simulink model "joystick"  (R2015a)
settings: Solver=ode45  StartTime=0.0  StopTime=inf  RelTol=1e-3
libraries: simulink x8, vrlib x1
settings Model: Creator=Trung Duc  LastModifiedBy=theth

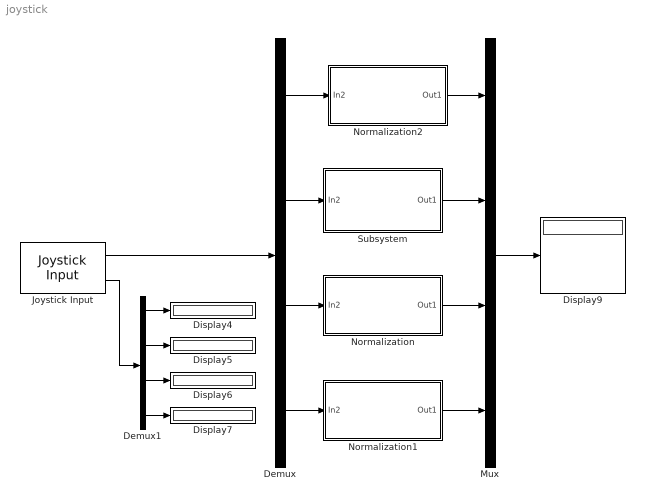
== system joystick ==
  Demux : Demux
  Demux1 : Demux
  Display{4..7,9} (5 alike) : Display
  Joystick Input : vrlib/Joystick Input  joyid=1  adjustports=on  forcefeed=off
  Mux : Mux
  Normalization : Subsystem
  Normalization1 : Subsystem
  Normalization2 : Subsystem
  Subsystem : Subsystem
  wires:
  Joystick Input/1 -> Demux/1
  Demux/1 -> Normalization2/1(In2)
  Demux1/1 -> Display4/1
  Demux1/2 -> Display5/1
  Demux1/3 -> Display6/1
  Demux1/4 -> Display7/1
  Joystick Input/2 -> Demux1/1
  Normalization2/1(Out1) -> Mux/1
  Normalization1/1(Out1) -> Mux/4
  Mux/1 -> Display9/1
  Demux/3 -> Normalization/1(In2)
  Normalization/1(Out1) -> Mux/3
  Demux/4 -> Normalization1/1(In2)
  Demux/2 -> Subsystem/1(In2)
  Subsystem/1(Out1) -> Mux/2

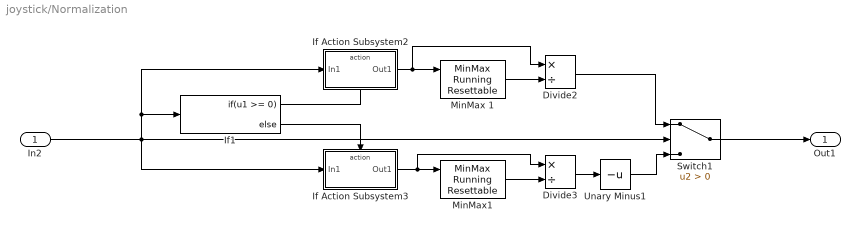
== system joystick/Normalization ==
  In2 : Inport
  Divide2 : Product  Inputs=*/
  Divide3 : Product  Inputs=*/
  If Action Subsystem2 : Subsystem  TreatAsAtomicUnit=on
  If Action Subsystem3 : Subsystem  TreatAsAtomicUnit=on
  If1 : If  IfExpression=u1 >= 0
  MinMax 1 : simulink/Math Operations/MinMax Running Resettable  Function=max  vinit=0.0
  MinMax1 : simulink/Math Operations/MinMax Running Resettable  Function=min  vinit=0.0
  Switch1 : Switch  Criteria=u2 > Threshold
  Unary Minus1 : UnaryMinus
  Out1 : Outport
  wires:
  Divide2/1 -> Switch1/1
  MinMax 1/1 -> Divide2/2
  If Action Subsystem2/1(Out1) -> Divide2/1, MinMax 1/1
  If1/1 -> If Action Subsystem2/Action
  Switch1/1 -> Out1/1
  If Action Subsystem3/1(Out1) -> MinMax1/1, Divide3/1
  MinMax1/1 -> Divide3/2
  In2/1 -> If Action Subsystem3/1(In1), Switch1/2, If Action Subsystem2/1(In1), If1/1
  Unary Minus1/1 -> Switch1/3
  Divide3/1 -> Unary Minus1/1
  If1/2 -> If Action Subsystem3/Action

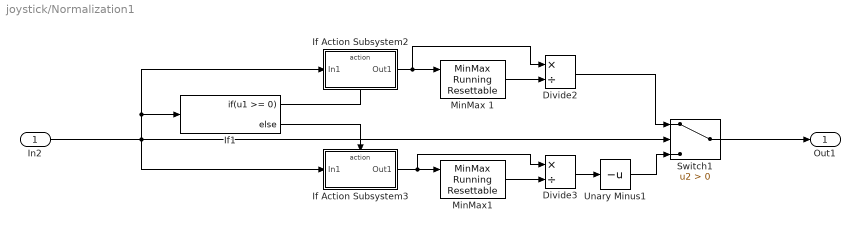
== system joystick/Normalization1 ==
  In2 : Inport
  Divide2 : Product  Inputs=*/
  Divide3 : Product  Inputs=*/
  If Action Subsystem2 : Subsystem  TreatAsAtomicUnit=on
  If Action Subsystem3 : Subsystem  TreatAsAtomicUnit=on
  If1 : If  IfExpression=u1 >= 0
  MinMax 1 : simulink/Math Operations/MinMax Running Resettable  Function=max  vinit=0.0
  MinMax1 : simulink/Math Operations/MinMax Running Resettable  Function=min  vinit=0.0
  Switch1 : Switch  Criteria=u2 > Threshold
  Unary Minus1 : UnaryMinus
  Out1 : Outport
  wires:
  Divide2/1 -> Switch1/1
  MinMax 1/1 -> Divide2/2
  If Action Subsystem2/1(Out1) -> Divide2/1, MinMax 1/1
  If1/1 -> If Action Subsystem2/Action
  Switch1/1 -> Out1/1
  If Action Subsystem3/1(Out1) -> MinMax1/1, Divide3/1
  MinMax1/1 -> Divide3/2
  In2/1 -> If Action Subsystem3/1(In1), Switch1/2, If Action Subsystem2/1(In1), If1/1
  Unary Minus1/1 -> Switch1/3
  Divide3/1 -> Unary Minus1/1
  If1/2 -> If Action Subsystem3/Action

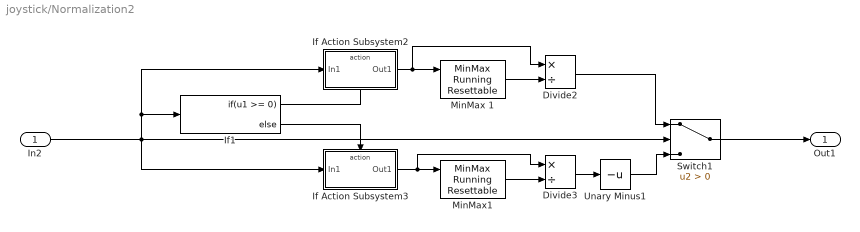
== system joystick/Normalization2 ==
  In2 : Inport
  Divide2 : Product  Inputs=*/
  Divide3 : Product  Inputs=*/
  If Action Subsystem2 : Subsystem  TreatAsAtomicUnit=on
  If Action Subsystem3 : Subsystem  TreatAsAtomicUnit=on
  If1 : If  IfExpression=u1 >= 0
  MinMax 1 : simulink/Math Operations/MinMax Running Resettable  Function=max  vinit=0.0
  MinMax1 : simulink/Math Operations/MinMax Running Resettable  Function=min  vinit=0.0
  Switch1 : Switch  Criteria=u2 > Threshold
  Unary Minus1 : UnaryMinus
  Out1 : Outport
  wires:
  Divide2/1 -> Switch1/1
  MinMax 1/1 -> Divide2/2
  If Action Subsystem2/1(Out1) -> Divide2/1, MinMax 1/1
  If1/1 -> If Action Subsystem2/Action
  Switch1/1 -> Out1/1
  If Action Subsystem3/1(Out1) -> MinMax1/1, Divide3/1
  MinMax1/1 -> Divide3/2
  In2/1 -> If Action Subsystem3/1(In1), Switch1/2, If Action Subsystem2/1(In1), If1/1
  Unary Minus1/1 -> Switch1/3
  Divide3/1 -> Unary Minus1/1
  If1/2 -> If Action Subsystem3/Action

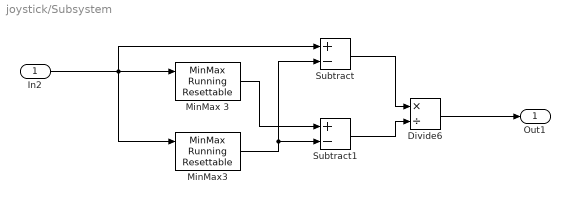
== system joystick/Subsystem ==
  In2 : Inport
  Divide6 : Product  Inputs=*/
  MinMax 3 : simulink/Math Operations/MinMax Running Resettable  Function=max  vinit=0.0
  MinMax3 : simulink/Math Operations/MinMax Running Resettable  Function=min  vinit=0.0
  Subtract : Sum  Inputs=+-
  Subtract1 : Sum  Inputs=+-
  Out1 : Outport
  wires:
  MinMax 3/1 -> Subtract1/1
  Subtract1/1 -> Divide6/2
  Divide6/1 -> Out1/1
  MinMax3/1 -> Subtract/2, Subtract1/2
  Subtract/1 -> Divide6/1
  In2/1 -> MinMax 3/1, MinMax3/1, Subtract/1

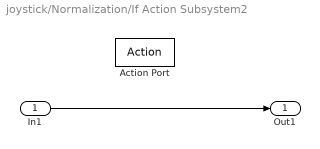
== system joystick/Normalization/If Action Subsystem2 ==
  In1 : Inport
  Action Port : ActionPort  ActionType=then
  Out1 : Outport
  wires:
  In1/1 -> Out1/1

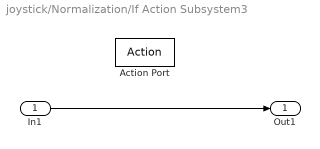
== system joystick/Normalization/If Action Subsystem3 ==
  In1 : Inport
  Action Port : ActionPort  ActionType=else
  Out1 : Outport
  wires:
  In1/1 -> Out1/1

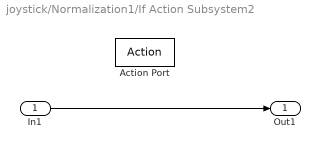
== system joystick/Normalization1/If Action Subsystem2 ==
  In1 : Inport
  Action Port : ActionPort
  Out1 : Outport
  wires:
  In1/1 -> Out1/1

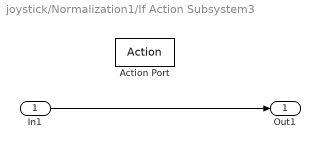
== system joystick/Normalization1/If Action Subsystem3 ==
  In1 : Inport
  Action Port : ActionPort
  Out1 : Outport
  wires:
  In1/1 -> Out1/1

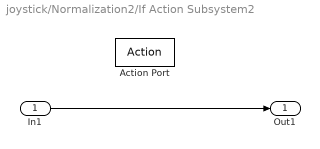
== system joystick/Normalization2/If Action Subsystem2 ==
  In1 : Inport
  Action Port : ActionPort
  Out1 : Outport
  wires:
  In1/1 -> Out1/1

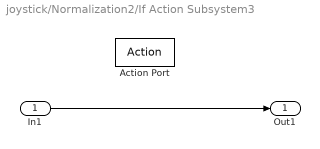
== system joystick/Normalization2/If Action Subsystem3 ==
  In1 : Inport
  Action Port : ActionPort
  Out1 : Outport
  wires:
  In1/1 -> Out1/1
